simulink model "embeddedM_example"  (R2018b)
settings: Solver=FixedStepDiscrete  StartTime=0.0  StopTime=10.0  RelTol=1e-3
undefined symbols (not defined in the file): C, N, Q, sysd
libraries: simulink x1
settings Model: Creator=wolfgang  LastModifiedBy=bigalfa
settings DebuggingCC: LibraryContextMissingDiagnostic=none
settings SFSimCC: SimUseLocalCustomCode=off
settings RTWCC: RTWUseLocalCustomCode=off

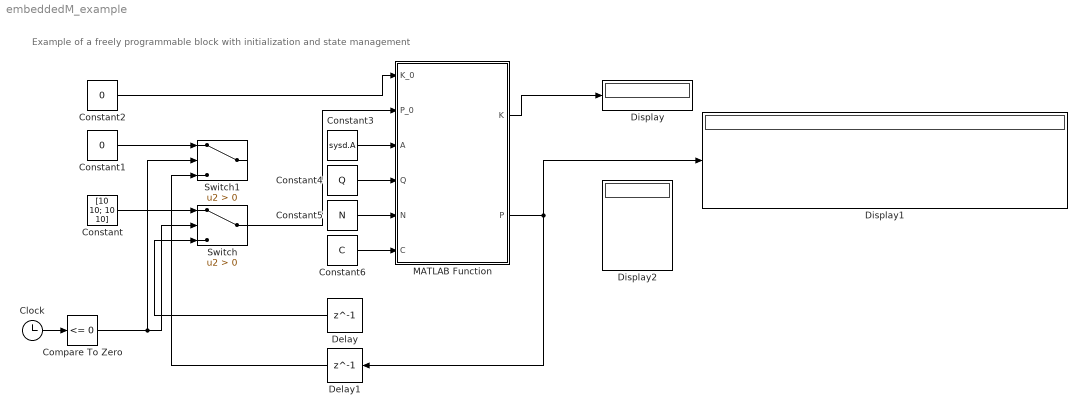
== system embeddedM_example ==
  note: Example of a freely programmable block with initialization and state management
  Clock : Clock
  Compare To Zero : simulink/Logic and Bit Operations/Compare To Zero  relop=<=  OutDataTypeStr=boolean
  Constant : Constant  Value=[10 10; 10 10]
  Constant1 : Constant  Value=0
  Constant2 : Constant  Value=0
  Constant3 : Constant  Value=sysd.A
  Constant4 : Constant  Value=Q
  Constant5 : Constant  Value=N
  Constant6 : Constant  Value=C
  Delay : Delay  DelayLength=1  InitialCondition=0  SampleTime=1
  Delay1 : Delay  DelayLength=1  InitialCondition=0  SampleTime=1
  Display : Display
  Display1 : Display
  Display2 : Display
  MATLAB Function : MATLAB Function  TreatAsAtomicUnit=on
  Switch : Switch  Criteria=u2 > Threshold
  Switch1 : Switch  Criteria=u2 > Threshold
  wires:
  MATLAB Function/2(P) -> Display1/1, Delay1/1
  Switch/1 -> MATLAB Function/2(P_0)
  Delay/1 -> Switch/3
  Constant/1 -> Switch/1
  Clock/1 -> Compare To Zero/1
  Compare To Zero/1 -> Switch1/2, Switch/2
  Constant1/1 -> Switch1/1
  Delay1/1 -> Switch1/3
  Constant2/1 -> MATLAB Function/1(K_0)
  MATLAB Function/1(K) -> Display/1
  Constant3/1 -> MATLAB Function/3(A)
  Constant4/1 -> MATLAB Function/4(Q)
  Constant5/1 -> MATLAB Function/5(N)
  Constant6/1 -> MATLAB Function/6(C)

== matlab function embeddedM_example/MATLAB Function ==
  data: K_0 input; K output; P_0 input; P output; A input; Q input; N input; C input


function [K,P] = fcn(K_0,P_0,A,Q,N,C)
P_1 = A * P_0 * A' + N*Q*N';
K = P_1*C'\(C*P_1*C'+R);
P = P_1 - K*C*P_1;
